simulink model "sampleModel1397"  (R2023a)
settings: Solver=VariableStepAuto  StartTime=0.0  StopTime=10.0  RelTol=1e-3
libraries: hdlsllib x5, simulink x2
settings Model: Creator=user1  LastModifiedBy=user1

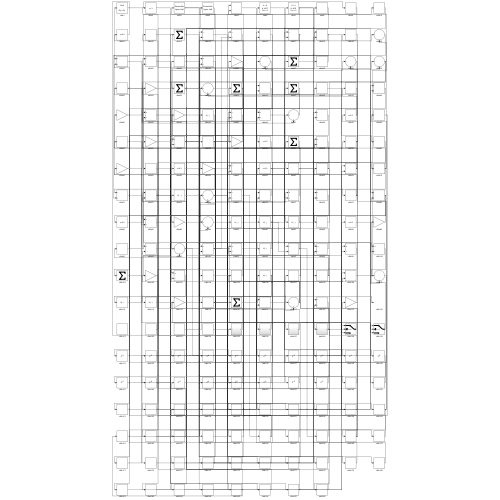
[thumbnail: Simulink's stored preview of the top-level diagram]
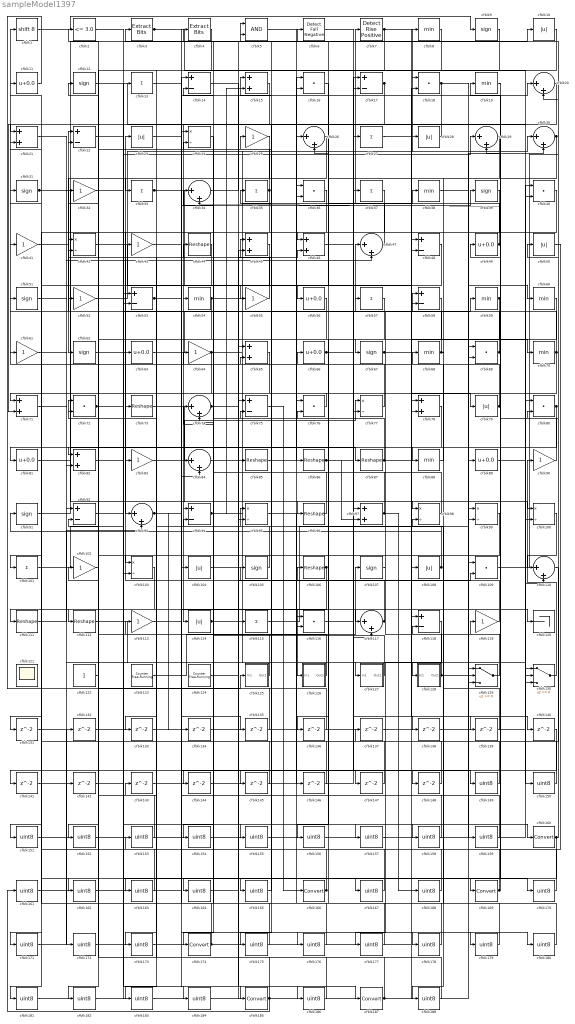
== system sampleModel1397 ==
  cfblk1 : ArithShift  BitShiftNumber=8
  cfblk{10,23,28,50,79,104,108,114} (8 alike) : Abs  SaturateOnIntegerOverflow=off
  cfblk{24,42,77,95,98..100,103} (8 alike) : Product  Inputs=*/  RndMeth=Zero  SaturateOnIntegerOverflow=on
  cfblk{13,27,33,35,37,57,101,115} (8 alike) : Sum  Inputs=+
  cfblk{25,32,41,43,52,55,61,64,83,90,102,113,119} (13 alike) : Gain
  cfblk{9,12,31,39,51,62,67,91,105,107} (10 alike) : Signum
  cfblk{44,73,85..87,96,106,111..112} (9 alike) : Reshape
  cfblk{16,18,36,40,69,72,76,80,109,116} (10 alike) : DotProduct  OutDataTypeStr=Inherit: Inherit via internal rule
  cfblk{11,49,56,63,66,81,89} (7 alike) : Bias  Bias=0.0  SaturateOnIntegerOverflow=off
  cfblk{20,26,29..30,34,47,74,84,93,110,117} (11 alike) : Sum  Inputs=|++
  cfblk{14,17,22,48,53,58,75,92,94,118} (10 alike) : Sum  Inputs=+-
  cfblk120 : Terminator
  cfblk121 : Scope
      settings: Floating=on
  cfblk122 : Constant  SampleTime=-1
  cfblk123 : hdlsllib/Sources/Counter Free-Running  NumBits=16  tsamp=-1
  cfblk124 : hdlsllib/Sources/Counter Free-Running  NumBits=16  tsamp=-1
  cfblk125 : Subsystem
      settings: LibrarySourceBlock=|
      | hdlsllib/Ports &
      | Subsystems/Subsystem
  cfblk126 : Subsystem
      settings: LibrarySourceBlock=|
      | hdlsllib/Ports &
      | Subsystems/Subsystem
  cfblk127 : Subsystem
      settings: LibrarySourceBlock=|
      | hdlsllib/Ports &
      | Subsystems/Subsystem
  cfblk128 : Subsystem
      settings: LibrarySourceBlock=|
      | hdlsllib/Ports &
      | Subsystems/Subsystem
  cfblk129 : Switch  SaturateOnIntegerOverflow=off  InputSameDT=off
  cfblk130 : Switch  SaturateOnIntegerOverflow=off  InputSameDT=off
  cfblk{131..148} (18 alike) : Delay  SampleTime=1
  cfblk{149..159,161..165,167..168,170..173,175..184,186,188} (34 alike) : DataTypeConversion  OutDataTypeStr=uint8  SaturateOnIntegerOverflow=off  RndMeth=Floor
  cfblk{15,21,45..46,65,71,78,82,97} (9 alike) : Sum
  cfblk{160,166,169,174,185,187} (6 alike) : DataTypeConversion  SaturateOnIntegerOverflow=off  RndMeth=Floor
  cfblk{8,19,38,54,59..60,68,70,88} (9 alike) : MinMax
  cfblk2 : hdlsllib/Logic and Bit Operations/Compare To Constant  relop=<=  const=3.0  OutDataTypeStr=boolean
  cfblk3 : simulink/Logic and Bit Operations/Extract Bits  bitsToExtract=Upper half  numBits=8  bitIdxRange=[0 7]  outScalingMode=Preserve fixed-point scaling
      settings: LibrarySourceBlock=|
      | hdlsllib/Logic and Bit
      | Operations/Extract Bits
  cfblk4 : simulink/Logic and Bit Operations/Extract Bits  bitsToExtract=Upper half  numBits=8  bitIdxRange=[0 7]  outScalingMode=Preserve fixed-point scaling
      settings: LibrarySourceBlock=|
      | hdlsllib/Logic and Bit
      | Operations/Extract Bits
  cfblk5 : Logic  AllPortsSameDT=off  OutDataTypeStr=boolean
  cfblk6 : hdlsllib/Logic and Bit Operations/Detect Fall Negative  vinit=0  OutDataTypeStr=boolean
  cfblk7 : hdlsllib/Logic and Bit Operations/Detect Rise Positive  vinit=0  OutDataTypeStr=boolean
  wires:
  cfblk52/1 -> cfblk30/1
  cfblk81/1 -> cfblk87/1
  cfblk79/1 -> cfblk1/1, cfblk5/2
  cfblk66/1 -> cfblk138/1, cfblk139/1
  cfblk128/1(Out1) -> cfblk95/1, cfblk30/2, cfblk148/1
  cfblk77/1 -> cfblk31/1
  cfblk109/1 -> cfblk3/1
  cfblk123/1 -> cfblk107/1
  cfblk76/1 -> cfblk71/1
  cfblk28/1 -> cfblk21/1
  cfblk106/1 -> cfblk126/1(In1), cfblk162/1
  cfblk64/1 -> cfblk59/1, cfblk173/1
  cfblk57/1 -> cfblk67/1
  cfblk27/1 -> cfblk8/1
  cfblk83/1 -> cfblk77/1
  cfblk119/1 -> cfblk23/1
  cfblk104/1 -> cfblk127/1(In1)
  cfblk36/1 -> cfblk93/1
  cfblk44/1 -> cfblk81/1
  cfblk11/1 -> cfblk125/1(In1)
  cfblk7/1 -> cfblk130/3, cfblk133/1, cfblk140/1
  cfblk19/1 -> cfblk169/1
  cfblk18/1 -> cfblk114/1, cfblk60/1
  cfblk130/1 -> cfblk90/1
  cfblk25/1 -> cfblk54/1
  cfblk47/1 -> cfblk7/1
  cfblk94/1 -> cfblk38/1, cfblk117/1, cfblk15/2
  cfblk59/1 -> cfblk29/2, cfblk183/1
  cfblk4/1 -> cfblk83/1
  cfblk1/1 -> cfblk9/1
  cfblk5/1 -> cfblk86/1
  cfblk91/1 -> cfblk5/1
  cfblk54/1 -> cfblk28/1, cfblk130/2, cfblk82/1, cfblk179/1
  cfblk73/1 -> cfblk100/1
  cfblk41/1 -> cfblk22/1
  cfblk16/1 -> cfblk56/1
  cfblk90/1 -> cfblk49/1
  cfblk49/1 -> cfblk6/1, cfblk34/2
  cfblk3/1 -> cfblk80/1, cfblk120/1
  cfblk68/1 -> cfblk47/1, cfblk188/1
  cfblk10/1 -> cfblk112/1
  cfblk97/1 -> cfblk45/1, cfblk168/1
  cfblk31/1 -> cfblk96/1, cfblk47/2
  cfblk26/1 -> cfblk62/1
  cfblk24/1 -> cfblk174/1
  cfblk88/1 -> cfblk68/1
  cfblk113/1 -> cfblk39/1
  cfblk86/1 -> cfblk27/1, cfblk97/2
  cfblk126/1(Out1) -> cfblk73/1
  cfblk17/1 -> cfblk55/1, cfblk165/1
  cfblk69/1 -> cfblk41/1, cfblk25/1
  cfblk2/1 -> cfblk129/2
  cfblk61/1 -> cfblk128/1(In1)
  cfblk70/1 -> cfblk22/2, cfblk50/1, cfblk175/1
  cfblk42/1 -> cfblk115/1
  cfblk82/1 -> cfblk29/1
  cfblk105/1 -> cfblk72/1
  cfblk72/1 -> cfblk58/1, cfblk155/1
  cfblk33/1 -> cfblk108/1, cfblk18/1
  cfblk9/1 -> cfblk33/1
  cfblk112/1 -> cfblk129/3
  cfblk37/1 -> cfblk103/1
  cfblk84/1 -> cfblk160/1
  cfblk21/1 -> cfblk92/1
  cfblk111/1 -> cfblk93/2
  cfblk67/1 -> cfblk70/1, cfblk79/1
  cfblk96/1 -> cfblk51/1
  cfblk55/1 -> cfblk42/1
  cfblk6/1 -> cfblk97/1
  cfblk98/1 -> cfblk44/1
  cfblk129/1 -> cfblk66/1
  cfblk100/1 -> cfblk110/1
  cfblk92/1 -> cfblk98/1
  cfblk35/1 -> cfblk2/1, cfblk74/2, cfblk82/2
  cfblk117/1 -> cfblk35/1, cfblk106/1, cfblk15/1
  cfblk115/1 -> cfblk89/1
  cfblk107/1 -> cfblk57/1
  cfblk85/1 -> cfblk16/1
  cfblk53/1 -> cfblk104/1, cfblk20/1, cfblk178/1
  cfblk63/1 -> cfblk37/1
  cfblk56/1 -> cfblk94/1
  cfblk48/1 -> cfblk101/1
  cfblk29/1 -> cfblk88/1
  cfblk8/1 -> cfblk17/2
  cfblk75/1 -> cfblk166/1
  cfblk22/1 -> cfblk103/2
  cfblk87/1 -> cfblk48/1, cfblk4/1
  cfblk43/1 -> cfblk187/1
  cfblk30/1 -> cfblk46/1, cfblk77/2
  cfblk122/1 -> cfblk52/1
  cfblk125/1(Out1) -> cfblk12/1
  cfblk93/1 -> cfblk134/1, cfblk135/1
  cfblk127/1(Out1) -> cfblk64/1
  cfblk101/1 -> cfblk63/1
  cfblk15/1 -> cfblk71/2
  cfblk114/1 -> cfblk109/2, cfblk58/2, cfblk186/1
  cfblk12/1 -> cfblk110/2
  cfblk108/1 -> cfblk91/1, cfblk34/1
  cfblk34/1 -> cfblk10/1
  cfblk32/1 -> cfblk185/1
  cfblk46/1 -> cfblk100/2
  cfblk74/1 -> cfblk46/2, cfblk176/1
  cfblk80/1 -> cfblk111/1, cfblk144/1
  cfblk103/1 -> cfblk131/1
  cfblk131/1 -> cfblk26/1
  cfblk132/1 -> cfblk69/2
  cfblk134/1 -> cfblk45/2
  cfblk135/1 -> cfblk92/2
  cfblk58/1 -> cfblk136/1
  cfblk136/1 -> cfblk94/2
  cfblk110/1 -> cfblk137/1
  cfblk137/1 -> cfblk130/1
  cfblk138/1 -> cfblk129/1
  cfblk139/1 -> cfblk98/2
  cfblk39/1 -> cfblk141/1
  cfblk141/1 -> cfblk53/2
  cfblk71/1 -> cfblk142/1
  cfblk143/1 -> cfblk16/2
  cfblk144/1 -> cfblk117/2
  cfblk20/1 -> cfblk145/1
  cfblk145/1 -> cfblk42/2
  cfblk95/1 -> cfblk146/1
  cfblk146/1 -> cfblk74/1
  cfblk23/1 -> cfblk147/1
  cfblk147/1 -> cfblk17/1
  cfblk148/1 -> cfblk61/1
  cfblk116/1 -> cfblk149/1
  cfblk149/1 -> cfblk26/2
  cfblk89/1 -> cfblk150/1
  cfblk150/1 -> cfblk116/1
  cfblk140/1 -> cfblk151/1
  cfblk151/1 -> cfblk116/2
  cfblk102/1 -> cfblk152/1
  cfblk152/1 -> cfblk36/2
  cfblk50/1 -> cfblk153/1
  cfblk153/1 -> cfblk102/1
  cfblk40/1 -> cfblk154/1
  cfblk154/1 -> cfblk36/1
  cfblk155/1 -> cfblk40/1
  cfblk60/1 -> cfblk156/1
  cfblk156/1 -> cfblk40/2
  cfblk14/1 -> cfblk157/1
  cfblk157/1 -> cfblk69/1
  cfblk133/1 -> cfblk158/1
  cfblk158/1 -> cfblk14/1
  cfblk38/1 -> cfblk159/1
  cfblk159/1 -> cfblk14/2
  cfblk160/1 -> cfblk20/2, cfblk80/2, cfblk181/1
  cfblk161/1 -> cfblk84/1
  cfblk162/1 -> cfblk84/2
  cfblk65/1 -> cfblk163/1
  cfblk163/1 -> cfblk72/2
  cfblk45/1 -> cfblk164/1
  cfblk164/1 -> cfblk65/1
  cfblk165/1 -> cfblk65/2
  cfblk166/1 -> cfblk105/1, cfblk11/1
  cfblk124/1 -> cfblk167/1
  cfblk167/1 -> cfblk75/1
  cfblk168/1 -> cfblk75/2
  cfblk169/1 -> cfblk109/1, cfblk119/1, cfblk53/1
  cfblk62/1 -> cfblk170/1
  cfblk170/1 -> cfblk19/1
  cfblk78/1 -> cfblk171/1
  cfblk171/1 -> cfblk132/1
  cfblk51/1 -> cfblk172/1
  cfblk172/1 -> cfblk78/1
  cfblk173/1 -> cfblk78/2
  cfblk174/1 -> cfblk95/2, cfblk18/2, cfblk21/2
  cfblk175/1 -> cfblk24/1
  cfblk176/1 -> cfblk24/2
  cfblk118/1 -> cfblk177/1
  cfblk177/1 -> cfblk76/2
  cfblk178/1 -> cfblk118/1
  cfblk179/1 -> cfblk118/2
  cfblk13/1 -> cfblk180/1
  cfblk180/1 -> cfblk76/1
  cfblk181/1 -> cfblk13/1
  cfblk99/1 -> cfblk182/1
  cfblk182/1 -> cfblk85/1
  cfblk183/1 -> cfblk99/1
  cfblk142/1 -> cfblk184/1
  cfblk184/1 -> cfblk99/2
  cfblk185/1 -> cfblk161/1, cfblk143/1
  cfblk186/1 -> cfblk32/1
  cfblk187/1 -> cfblk48/2, cfblk113/1
  cfblk188/1 -> cfblk43/1

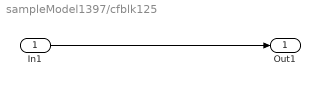
== system sampleModel1397/cfblk125 ==
  In1 : Inport
  Out1 : Outport
  wires:
  In1/1 -> Out1/1

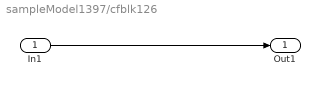
== system sampleModel1397/cfblk126 ==
  In1 : Inport
  Out1 : Outport
  wires:
  In1/1 -> Out1/1

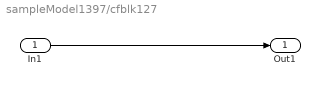
== system sampleModel1397/cfblk127 ==
  In1 : Inport
  Out1 : Outport
  wires:
  In1/1 -> Out1/1

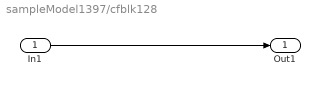
== system sampleModel1397/cfblk128 ==
  In1 : Inport
  Out1 : Outport
  wires:
  In1/1 -> Out1/1
